simulink model "Cell_modelling_and_control"  (R2019b)
settings: Solver=VariableStepAuto  StartTime=0.0  StopTime=900  MaxStep=0.01  RelTol=1e-3
settings Model: Creator=matm  LastModifiedBy=jorge
settings SolverCC: ShapePreserveControl=EnableAll  SolverResetMethod=Robust
settings DataIOCC: ReturnWorkspaceOutputs=off
settings DebuggingCC: ArithmeticOperatorsInVariantConditions=warning
settings SFSimCC: SimUseLocalCustomCode=off  CustomCodeUndefinedFunction=UseInterfaceOnly
settings RTWCC: RTWUseLocalCustomCode=off
settings CodeAppCC: StateflowObjectComments=on

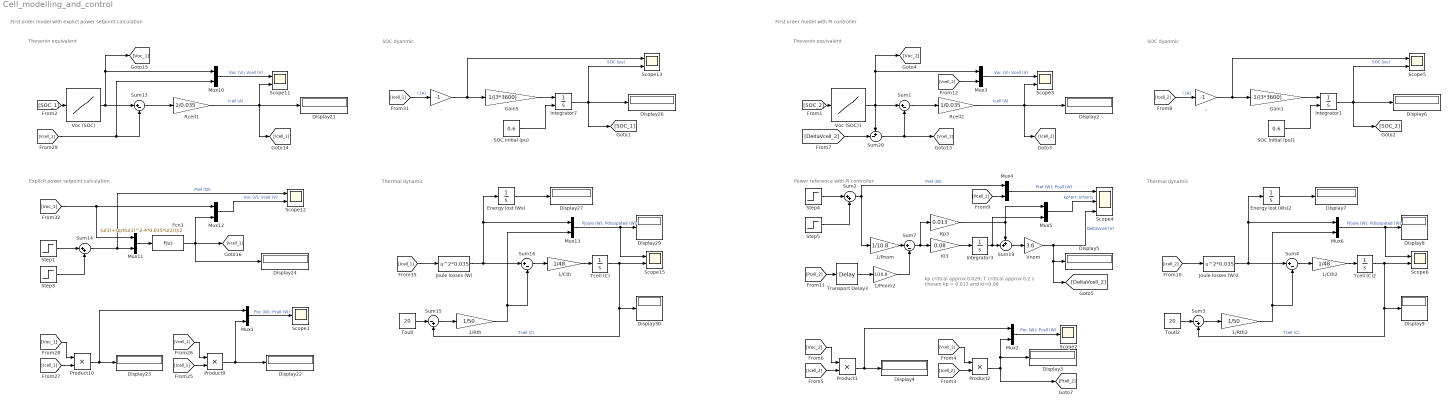
== system Cell_modelling_and_control ==
  note: Thermal dynamic
  note: Explicit power setpoint calculation
  note: SOC dyanmic
  note: Thevenin equivalent
  note: First order model with explict power setpoint calculation
  note: SOC dyanmic
  note: Thevenin equivalent
  note: Thermal dynamic
  note: Power reference with PI controller
  note: First order model with PI controller
  note: kp critical approx 0.029; T critical approx 0.2 s
      | chosen kp = 0.013 and ki=0.08
  . : Gain  Gain=-1
  .. : Gain  Gain=-1
  1/Cth : Gain  Gain=1/48
  1/Cth2 : Gain  Gain=1/48
  1/Pnom : Gain  Gain=1/10.8
  1/Pnom2 : Gain  Gain=1/10.8
  1/Rth : Gain  Gain=1/50
  1/Rth2 : Gain  Gain=1/50
  Display{2..9,21..24,26..27,29..30} (16 alike) : Display
  Energy lost (Ws) : Integrator  ZeroCross=off
  Energy lost (Ws)2 : Integrator  ZeroCross=off
  Fcn1 : Fcn  Expr=(u(1)+sqrt(u(1)^2-4*0.035*u(2)))/2
  Gain1 : Gain  Gain=1/(3*3600)
  Gain5 : Gain  Gain=1/(3*3600)
  Integrator1 : Integrator  InitialConditionSource=external  InitialCondition=0.5  ZeroCross=off
  Integrator3 : Integrator  ZeroCross=off
  Integrator7 : Integrator  InitialConditionSource=external  InitialCondition=0.5  ZeroCross=off
  Joule losses (W) : Fcn  Expr=u^2*0.035
  Joule losses (W)2 : Fcn  Expr=u^2*0.035
  Ki3 : Gain  Gain=0.08
  Kp3 : Gain  Gain=0.013
  Mux{1..6,10..13} (10 alike) : Mux  Inputs=2
  Product{1..2,9..10} (4 alike) : Product
  Rcell1 : Gain  Gain=1/0.035
  Rcell2 : Gain  Gain=1/0.035
  SOC initial (pu) : Constant  Value=0.6
  SOC initial (pu)1 : Constant  Value=0.6
  Scope1 : Scope
  Scope{3,5..6,11..13,15} (7 alike) : Scope  NumInputPorts=2
  Scope2 : Scope
  Scope4 : Scope  NumInputPorts=3
  Step1 : Step  Time=10  After=20  SampleTime=0
  Step3 : Step  Time=610  After=-20  SampleTime=0
  Step4 : Step  Time=10  After=20  SampleTime=0
  Step5 : Step  Time=610  After=-20  SampleTime=0
  Sum{1,4,7,13,16} (5 alike) : Sum  Inputs=|+-
  Sum14 : Sum  Inputs=|++
  Sum15 : Sum  Inputs=|-+
  Sum19 : Sum  Inputs=++|
  Sum2 : Sum  Inputs=|++
  Sum20 : Sum  Inputs=+-|
  Sum3 : Sum  Inputs=|-+
  Tcell (C) : Integrator  InitialCondition=20  ZeroCross=off
  Tcell (C)2 : Integrator  InitialCondition=20  ZeroCross=off
  Toutl : Constant  Value=20
  Toutl2 : Constant  Value=20
  Transport Delay3 : TransportDelay  DelayTime=0.1
  Vnom : Gain  Gain=3.6
  Voc (SOC) : Lookup_n-D  NumberOfTableDimensions=1  BreakpointsForDimension1=[0 0.1 0.2 0.3 0.4 0.5 0.6 0.7 0.8 0.9 1]  Table=[2.85 3.19 3.39 3.52 3.65 3.73 3.82 3.92 4.01 4.07 4.19]  InternalRulePriority=Speed  RndMeth=Simplest  InputSameDT=on
  Voc (SOC)1 : Lookup_n-D  NumberOfTableDimensions=1  BreakpointsForDimension1=[0 0.1 0.2 0.3 0.4 0.5 0.6 0.7 0.8 0.9 1]  Table=[2.85 3.19 3.39 3.52 3.65 3.73 3.82 3.92 4.01 4.07 4.19]  InternalRulePriority=Speed  RndMeth=Simplest  InputSameDT=on
  wires:
  Mux11/1 -> Fcn1/1
  [Voc_1] -> Product10/1
  Step1/1 -> Sum14/1
  Voc (SOC)/1 -> [Voc_1], Mux10/1, Sum13/1
  Rcell1/1 -> [Icell_1], Scope11/2, Display21/1  "Icell (A)"
  SOC initial (pu)/1 -> Integrator7/2
  Mux12/1 -> Scope12/2  "Voc (V); Vcell (V)"
  [Icell_1] -> ./1  "I (A)"
  Integrator7/1 -> [SOC_1], Scope13/2, Display26/1  "SOC (pu)"
  [Voc_1] -> Mux11/1, Mux12/1
  Sum14/1 -> Scope12/1, Mux11/2  "Pref (W)"
  Sum13/1 -> Rcell1/1
  Gain5/1 -> Integrator7/1
  Product9/1 -> Mux1/2, Display22/1
  [Icell_1] -> Product9/2
  [Vcell_1] -> Sum13/2, Mux10/2
  ./1 -> Scope13/1, Gain5/1
  Product10/1 -> Mux1/1, Display23/1
  [Vcell_1] -> Product9/1
  [Icell_1] -> Product10/2
  Mux10/1 -> Scope11/1  "Voc (V); Vcell (V)"
  Fcn1/1 -> Mux12/2, [Vcell_1], Display24/1
  Energy lost (Ws)/1 -> Display27/1
  1/Cth/1 -> Tcell (C)/1
  Mux13/1 -> Display29/1, Scope15/1  "Pjoule (W); Pdissipated (W)"
  [Icell_1] -> Joule losses (W)/1
  Toutl/1 -> Sum15/1
  Tcell (C)/1 -> Scope15/2, Display30/1, Sum15/2  "Tcell (C)"
  Sum16/1 -> 1/Cth/1
  1/Rth/1 -> Sum16/2, Mux13/2
  Sum15/1 -> 1/Rth/1
  Joule losses (W)/1 -> Sum16/1, Energy lost (Ws)/1, Mux13/1
  [SOC_1] -> Voc (SOC)/1
  Mux1/1 -> Scope1/1  "Poc (W); Pcell (W)"
  Voc (SOC)1/1 -> [Voc_2], Mux3/1, Sum20/1, Sum1/1
  [SOC_2] -> Voc (SOC)1/1
  Integrator1/1 -> [SOC_2], Scope5/2, Display6/1  "SOC (pu)"
  Mux6/1 -> Display8/1, Scope6/1  "Pjoule (W); Pdissipated (W)"
  Joule losses (W)2/1 -> Sum4/1, Energy lost (Ws)2/1, Mux6/1
  1/Rth2/1 -> Sum4/2, Mux6/2
  Sum4/1 -> 1/Cth2/1
  Sum3/1 -> 1/Rth2/1
  Mux2/1 -> Scope2/1  "Poc (W); Pcell (W)"
  [Icell_2] -> Joule losses (W)2/1
  Tcell (C)2/1 -> Scope6/2, Display9/1, Sum3/2  "Tcell (C)"
  Mux3/1 -> Scope3/1  "Voc (V); Vcell (V)"
  Energy lost (Ws)2/1 -> Display7/1
  1/Cth2/1 -> Tcell (C)2/1
  [Icell_2] -> Product1/2
  [Vcell_2] -> Product2/1
  Sum1/1 -> Rcell2/1
  Product1/1 -> Mux2/1, Display4/1
  Step4/1 -> Sum2/1
  Gain1/1 -> Integrator1/1
  Product2/1 -> Mux2/2, Display3/1, [Pcell_2]
  [Icell_2] -> Product2/2
  ../1 -> Scope5/1, Gain1/1
  Toutl2/1 -> Sum3/1
  Sum2/1 -> Mux4/1, 1/Pnom/1  "Pref (W)"
  [Voc_2] -> Product1/1
  SOC initial (pu)1/1 -> Integrator1/2
  Rcell2/1 -> [Icell_2], Scope3/2, Display2/1  "Icell (A)"
  [Icell_2] -> ../1  "I (A)"
  Step3/1 -> Sum14/2
  Step5/1 -> Sum2/2
  1/Pnom/1 -> Sum7/1
  1/Pnom2/1 -> Sum7/2
  Transport Delay3/1 -> 1/Pnom2/1
  [Pcell_2] -> Transport Delay3/1
  Sum7/1 -> Kp3/1, Ki3/1
  Ki3/1 -> Integrator3/1
  Integrator3/1 -> Mux5/2, Sum19/2
  Kp3/1 -> Mux5/1, Sum19/1
  Mux4/1 -> Scope4/1  "Pref (W); Pcell (W)"
  [Pcell_2] -> Mux4/2
  Mux5/1 -> Scope4/2  "kp*err; ki*err/s"
  Sum19/1 -> Vnom/1
  [DeltaVcell_2] -> Sum20/2
  Sum20/1 -> [Vcell_2], Sum1/2
  [Vcell_2] -> Mux3/2
  Vnom/1 -> Scope4/3, [DeltaVcell_2], Display5/1  "DeltaVcell (V)"
